simulink model "exnb4137986_Q8"  (R2024b)
settings: Solver=FixedStepAuto  StartTime=0.0  StopTime=5  FixedStep=0.001  RelTol=1e-3
values from neighbouring files (symbols this model uses):
  C = [0, 1]    [exnb4137986_Q10_par.m]    (also in exnb4137986_Q5_par.m = [C, A^i * B]; exnb4137986_Q7_par.m = [C, A^i * B]; exnb4137986_Q8_par.m = [0 1]; exnb4137986_Q9_par.m = jacobian(y, X))
  Ki = lqi(sys_CT,Q,R)    [exnb4137986_Q8_par.m]
  values = [0, 0.01, 1, 0.001, 1, 1, 10]    [exnb4137986_Q10_par.m]    (also in exnb4137986_Q4_par.m; exnb4137986_Q5_par.m; exnb4137986_Q7_par.m; exnb4137986_Q8_par.m)
  x_star_1 = [I_star_1, omega_star_1]    [exnb4137986_Q10_par.m]    (also in exnb4137986_Q4_par.m = [omega_star_1, I_star_1]; exnb4137986_Q5_par.m; exnb4137986_Q7_par.m; exnb4137986_Q8_par.m)
  x_star_2 = [0, 10]    [exnb4137986_Q10_par.m]    (also in exnb4137986_Q7_par.m; exnb4137986_Q8_par.m)
settings Model: Creator=therkelsen  LastModifiedBy=therkelsen

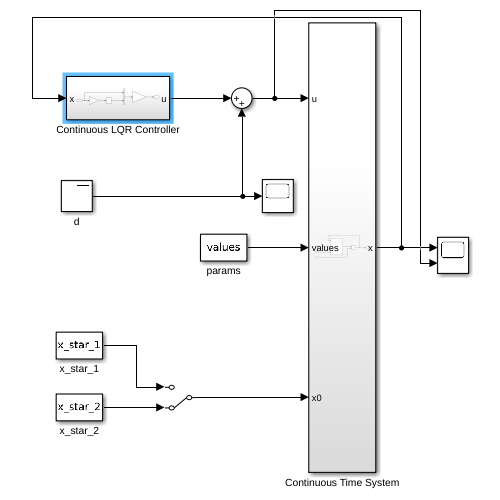
[thumbnail: Simulink's stored preview of the top-level diagram]
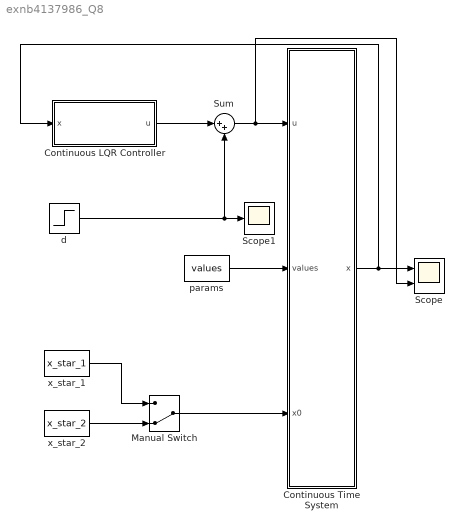
== system exnb4137986_Q8 ==
  Continuous LQR Controller : Subsystem
  Continuous Time System : Subsystem
  Manual Switch : ManualSwitch  CurrentSetting=0
  Scope : Scope  NumInputPorts=2
  Scope1 : Scope
  Sum : Sum  Inputs=|++
  d : Step  Time=2  After=5  SampleTime=0
  params : Constant  Value=values
  x_star_1 : Constant  Value=x_star_1
  x_star_2 : Constant  Value=x_star_2
  wires:
  Manual Switch/1 -> Continuous Time System/3(x0)
  Continuous LQR Controller/1(u) -> Sum/1
  params/1 -> Continuous Time System/2(values)
  x_star_2/1 -> Manual Switch/2
  x_star_1/1 -> Manual Switch/1
  d/1 -> Sum/2, Scope1/1
  Sum/1 -> Scope/2, Continuous Time System/1(u)
  Continuous Time System/1(x) -> Continuous LQR Controller/1(x), Scope/1

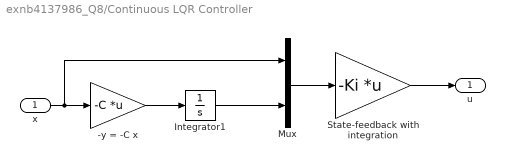
== system exnb4137986_Q8/Continuous LQR Controller ==
  x : Inport
  -y = -C x : Gain  Gain=-C  Multiplication=Matrix(K*u) (u vector)
  Integrator1 : Integrator
  Mux : Mux  Inputs=2
  State-feedback with integration : Gain  Gain=-Ki  Multiplication=Matrix(K*u) (u vector)
  u : Outport
  wires:
  x/1 -> Mux/1, -y = -C x/1
  -y = -C x/1 -> Integrator1/1
  Integrator1/1 -> Mux/2
  Mux/1 -> State-feedback with integration/1
  State-feedback with integration/1 -> u/1

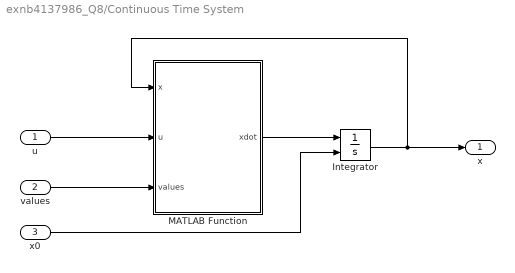
== system exnb4137986_Q8/Continuous Time System ==
  u : Inport
  values : Inport  Port=2
  x0 : Inport  Port=3
  Integrator : Integrator  InitialConditionSource=external
  MATLAB Function : MATLAB Function  TreatAsAtomicUnit=on
  x : Outport
  wires:
  MATLAB Function/1(xdot) -> Integrator/1
  values/1 -> MATLAB Function/3(values)
  u/1 -> MATLAB Function/2(u)
  Integrator/1 -> x/1, MATLAB Function/1(x)
  x0/1 -> Integrator/2

== matlab function exnb4137986_Q8/Continuous Time System/MATLAB Function ==
  data: x input; u input; xdot output; values input
function xdot = fcn(x, u, values)

J = values(2);
L = values(3);
Kd = values(4);
Ke = values(5);
Km = values(6);
Rm = values(7);

xdot = [-Rm/L * x(1) - Ke/L * x(2) + 1/L * u;
         Km/J * x(1) - Kd/J * x(2)];
